simulink model "TEST_IPM_2_0"  (R2019b)
settings: configuration reference "Configuration" (kept outside this file)
PreLoadFcn:
  | RTWConfigurationCB('preloadfcn', bdroot);
values from neighbouring files (symbols this model uses):
  MParamFbase = 200.0    [TEST_IPM_LIB.sldd]
  MParamIbase = 360.0    [TEST_IPM_LIB.sldd]
  MParamLd = 8.0E-5    [TEST_IPM_LIB.sldd]
  MParamLq = 0.00028    [TEST_IPM_LIB.sldd]
  MParamRs = 0.014    [TEST_IPM_LIB.sldd]
  PWM_TPBRD_HALF = 5000.0    [TEST_IPM_LIB.sldd]
  Ts_10kHz = 0.0001    [TEST_IPM_LIB.sldd]
  Ts_1kHz = 0.001    [TEST_IPM_LIB.sldd]
undefined symbols (not defined in the file or in its folder): DiscIntNeverNeededParam, Down, GPTRIP1SEL, GPTRIP2SEL, TZ1, TZ2, Up
libraries: c280xlib x24, c2837xDlib x18, dsparch4 x11, c2802xlib x10, powerlib_meascontrol x9, dspstat3 x2, c2000lib x1, c2806xlib x1, idelinklib_common x1
(part 5 of 6)

== system TEST_IPM_2_0/INT/Motor Control/SVPWM/Inverse Park Transformation ==
  D : Inport
  Q : Inport  Port=2
  theta : Inport  Port=3
  Product{,1..3} (4 alike) : Product  OutDataTypeStr=Inherit: Same as first input
  Sin : Trigonometry  OutputSignalType=real
  Sin1 : Trigonometry  Operator=cos  OutputSignalType=real
  Sum1 : Sum  Inputs=|++  OutDataTypeStr=Inherit: Same as first input
  Sum2 : Sum  Inputs=|+-  OutDataTypeStr=Inherit: Same as first input
  Alpha : Outport
  Beta : Outport  Port=2
  wires:
  Sin1/1 -> Product2/2, Product/2
  Sin/1 -> Product3/2, Product1/2
  Product3/1 -> Sum1/2
  Sum1/1 -> Beta/1
  D/1 -> Product3/1, Product/1
  Product2/1 -> Sum1/1
  Sum2/1 -> Alpha/1
  Product/1 -> Sum2/1
  Product1/1 -> Sum2/2
  Q/1 -> Product2/1, Product1/1
  theta/1 -> Sin/1, Sin1/1

== system TEST_IPM_2_0/INT/Motor Control/SpeedMode/Function-Call Subsystem ==
  function : TriggerPort  TriggerType=function-call  VariantControl=Variant
  Abs : Abs  Commented=on  OutDataTypeStr=single
  Constant : Constant  Value=0  OutDataTypeStr=single  SampleTime=-1
  Constant1 : Constant  Value=0  OutDataTypeStr=single  SampleTime=-1
  Constant2 : Constant  Value=0  OutDataTypeStr=single
  Data Store Read1 : DataStoreRead  DataStoreName=N_FBK
  Data Store Read2 : DataStoreRead  DataStoreName=STOP
  Data Store Read3 : DataStoreRead  DataStoreName=N_REF
  Data Store Write1 : DataStoreWrite  DataStoreName=Iq_REF
  Data Store Write2 : DataStoreWrite  DataStoreName=Id_REF
  Demux : Demux  Outputs=2
  Gain : Gain  Commented=on  Gain=-0.5  OutDataTypeStr=single
  Gain1 : Gain  Commented=on  Gain=0.866  OutDataTypeStr=single
  Mux : Mux  Inputs=2
  Mux1 : Mux  Inputs=2
  "PID_n " : Subsystem
  Switch : Switch  Criteria=u2 ~= 0
  wires:
  Constant/1 -> Mux1/1
  Constant1/1 -> Mux1/2
  Switch/1 -> Demux/1
  Data Store Read1/1 -> Mux/2
  Demux/2 -> "PID_n "/2(Fbk)
  Demux/1 -> "PID_n "/1(Ref)
  Mux1/1 -> Switch/1
  Data Store Read2/1 -> Switch/2
  Data Store Read3/1 -> Mux/1
  Mux/1 -> Switch/3
  "PID_n "/1(Out) -> Data Store Write1/1, Abs/1
  Abs/1 -> Gain/1
  Constant2/1 -> Data Store Write2/1

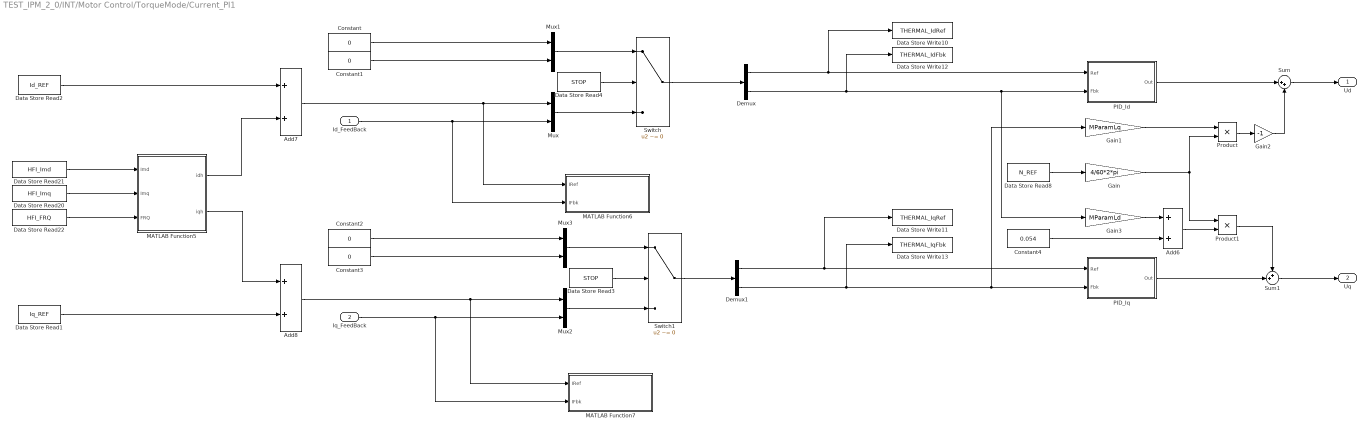
== system TEST_IPM_2_0/INT/Motor Control/TorqueMode/Current_PI1 ==
  Id_FeedBack : Inport
  Iq_FeedBack : Inport  Port=2
  Add6 : Sum
  Add7 : Sum
  Add8 : Sum
  Constant{,1..3} (4 alike) : Constant  Value=0  OutDataTypeStr=single  SampleTime=-1
  Constant4 : Constant  Value=0.054  OutDataTypeStr=single  SampleTime=-1
  Data Store Read1 : DataStoreRead  DataStoreName=Iq_REF
  Data Store Read2 : DataStoreRead  DataStoreName=Id_REF
  Data Store Read20 : DataStoreRead  DataStoreName=HFI_Imq
  Data Store Read21 : DataStoreRead  DataStoreName=HFI_Imd
  Data Store Read22 : DataStoreRead  DataStoreName=HFI_FRQ
  Data Store Read3 : DataStoreRead  DataStoreName=STOP
  Data Store Read4 : DataStoreRead  DataStoreName=STOP
  Data Store Read8 : DataStoreRead  DataStoreName=N_REF
  Data Store Write10 : DataStoreWrite  DataStoreName=THERMAL_IdRef
  Data Store Write11 : DataStoreWrite  DataStoreName=THERMAL_IqRef
  Data Store Write12 : DataStoreWrite  DataStoreName=THERMAL_IdFbk
  Data Store Write13 : DataStoreWrite  DataStoreName=THERMAL_IqFbk
  Demux : Demux  Outputs=2
  Demux1 : Demux  Outputs=2
  Gain : Gain  Gain=4/60*2*pi
  Gain1 : Gain  Gain=MParamLq
  Gain2 : Gain  Gain=-1
  Gain3 : Gain  Gain=MParamLd
  MATLAB Function5 : MATLAB Function  TreatAsAtomicUnit=on
  MATLAB Function6 : MATLAB Function  TreatAsAtomicUnit=on
  MATLAB Function7 : MATLAB Function  TreatAsAtomicUnit=on
  Mux{,1..3} (4 alike) : Mux  Inputs=2
  "PID_Id " : Subsystem  TreatAsAtomicUnit=on
  PID_Iq : Subsystem  TreatAsAtomicUnit=on
  Product : Product
  Product1 : Product
  Sum : Sum  Inputs=|++  AccumDataTypeStr=single
  Sum1 : Sum  Inputs=++|  AccumDataTypeStr=single
  Switch : Switch  Criteria=u2 ~= 0
  Switch1 : Switch  Criteria=u2 ~= 0
  Ud : Outport
  Uq : Outport  Port=2
  wires:
  Demux1/2 -> Data Store Write13/1, Gain1/1, PID_Iq/2(Fbk)
  Demux/1 -> Data Store Write10/1, "PID_Id "/1(Ref)
  Data Store Read1/1 -> Add8/2
  Add8/1 -> MATLAB Function7/1(IRef), Mux2/1
  Constant3/1 -> Mux3/2
  Gain2/1 -> Sum/2
  "PID_Id "/1(Out) -> Sum/1
  Gain/1 -> Product1/1, Product/2
  Switch/1 -> Demux/1
  Data Store Read21/1 -> MATLAB Function5/1(Imd)
  Mux3/1 -> Switch1/1
  Switch1/1 -> Demux1/1
  Gain3/1 -> Add6/1
  Mux/1 -> Switch/3
  Data Store Read3/1 -> Switch1/2
  Iq_FeedBack/1 -> MATLAB Function7/2(IFbk), Mux2/2
  Add6/1 -> Product1/2
  Gain1/1 -> Product/1
  Mux2/1 -> Switch1/3
  Data Store Read8/1 -> Gain/1
  Constant2/1 -> Mux3/1
  MATLAB Function5/1(idh) -> Add7/2
  MATLAB Function5/2(iqh) -> Add8/1
  Data Store Read20/1 -> MATLAB Function5/2(Imq)
  Constant1/1 -> Mux1/2
  Product1/1 -> Sum1/1
  Mux1/1 -> Switch/1
  Data Store Read4/1 -> Switch/2
  Constant4/1 -> Add6/2
  Add7/1 -> MATLAB Function6/1(IRef), Mux/1
  Data Store Read2/1 -> Add7/1
  PID_Iq/1(Out) -> Sum1/2
  Data Store Read22/1 -> MATLAB Function5/3(FRQ)
  Constant/1 -> Mux1/1
  Id_FeedBack/1 -> MATLAB Function6/2(IFbk), Mux/2
  Demux/2 -> Data Store Write12/1, Gain3/1, "PID_Id "/2(Fbk)
  Demux1/1 -> Data Store Write11/1, PID_Iq/1(Ref)
  Product/1 -> Gain2/1
  Sum/1 -> Ud/1
  Sum1/1 -> Uq/1

== system TEST_IPM_2_0/INT/Motor Control/TorqueMode/Function-Call Subsystem ==
  function : TriggerPort  TriggerType=function-call  VariantControl=Variant
  Constant : Constant  Value=0  OutDataTypeStr=single  SampleTime=-1
  Constant1 : Constant  Value=0  OutDataTypeStr=single  SampleTime=-1
  Constant2 : Constant  Value=0  OutDataTypeStr=single  SampleTime=-1
  Constant3 : Constant  OutDataTypeStr=uint16  SampleTime=-1
  Data Store Write : DataStoreWrite  DataStoreName=N_Integral
  Data Store Write1 : DataStoreWrite  DataStoreName=Iq_Integral
  Data Store Write2 : DataStoreWrite  DataStoreName=Id_Integral
  Data Store Write3 : DataStoreWrite  DataStoreName=REVERSE_FLAG
  wires:
  Constant1/1 -> Data Store Write2/1
  Constant2/1 -> Data Store Write1/1
  Constant/1 -> Data Store Write/1
  Constant3/1 -> Data Store Write3/1

== system TEST_IPM_2_0/INT/Motor Control/TorqueMode/PID_n  ==
  Ref : Inport
  Fbk : Inport  Port=2
  Constant : Constant  Value=40*1.2  OutDataTypeStr=single  SampleTime=-1
  Data Store Read : DataStoreRead  DataStoreName=Udc_Integral
  Data Store Read2 : DataStoreRead  DataStoreName=Udc_Kp
  Data Store Write1 : DataStoreWrite  DataStoreName=Udc_Integral
  MATLAB Function : MATLAB Function  TreatAsAtomicUnit=on
  Product : Product  OutDataTypeStr=Inherit: Same as first input
  Subsystem : Subsystem
  Sum1 : Sum  OutDataTypeStr=single
  Sum2 : Sum  Inputs=+-  OutDataTypeStr=Inherit: Inherit via back propagation
  Out : Outport
  wires:
  Data Store Read/1 -> Subsystem/1(OLD_UI_REG3)
  Fbk/1 -> Sum2/2
  Ref/1 -> Sum2/1
  Product/1 -> Sum1/1
  Data Store Read2/1 -> Product/2
  Subsystem/1(UI_REG1) -> Data Store Write1/1, Sum1/2
  Sum2/1 -> Subsystem/2(up_reg3), Product/1
  MATLAB Function/1(Output) -> Out/1
  Sum1/1 -> MATLAB Function/2(Input)
  Constant/1 -> MATLAB Function/1(Limit)

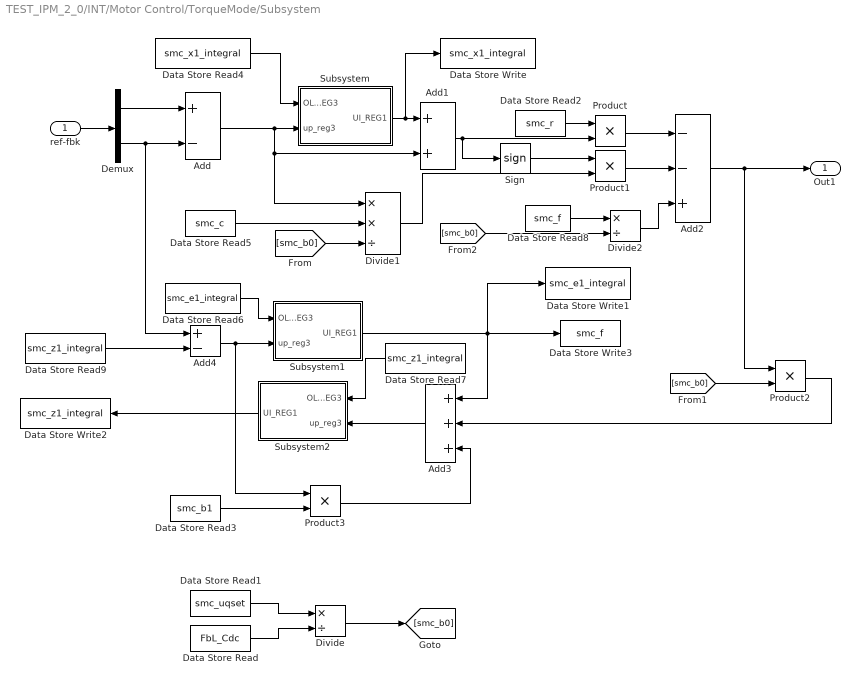
== system TEST_IPM_2_0/INT/Motor Control/TorqueMode/Subsystem ==
  ref-fbk : Inport
  Add : Sum  Inputs=+-
  Add1 : Sum
  Add2 : Sum  Inputs=--+
  Add3 : Sum  Inputs=+++
  Add4 : Sum  Inputs=+-
  Data Store Read : DataStoreRead  DataStoreName=FbL_Cdc
  Data Store Read1 : DataStoreRead  DataStoreName=smc_uqset
  Data Store Read2 : DataStoreRead  DataStoreName=smc_r
  Data Store Read3 : DataStoreRead  DataStoreName=smc_b1
  Data Store Read4 : DataStoreRead  DataStoreName=smc_x1_integral
  Data Store Read5 : DataStoreRead  DataStoreName=smc_c
  Data Store Read6 : DataStoreRead  DataStoreName=smc_e1_integral
  Data Store Read7 : DataStoreRead  DataStoreName=smc_z1_integral
  Data Store Read8 : DataStoreRead  DataStoreName=smc_f
  Data Store Read9 : DataStoreRead  DataStoreName=smc_z1_integral
  Data Store Write : DataStoreWrite  DataStoreName=smc_x1_integral
  Data Store Write1 : DataStoreWrite  DataStoreName=smc_e1_integral
  Data Store Write2 : DataStoreWrite  DataStoreName=smc_z1_integral
  Data Store Write3 : DataStoreWrite  DataStoreName=smc_f
  Demux : Demux  Outputs=2
  Divide : Product  Inputs=*/
  Divide1 : Product  Inputs=**/
  Divide2 : Product  Inputs=*/
  Product{,1..3} (4 alike) : Product
  Sign : Signum
  Subsystem : Subsystem
  Subsystem1 : Subsystem
  Subsystem2 : Subsystem
  Out1 : Outport
  wires:
  ref-fbk/1 -> Demux/1
  Demux/1 -> Add/1
  Demux/2 -> Add4/1, Add/2
  Add/1 -> Divide1/1, Add1/2, Subsystem/2(up_reg3)
  Subsystem/1(UI_REG1) -> Data Store Write/1, Add1/1
  Add1/1 -> Product/2, Sign/1
  Data Store Read2/1 -> Product/1
  Product/1 -> Add2/1
  Product1/1 -> Add2/2
  Sign/1 -> Product1/1
  Data Store Read1/1 -> Divide/1
  Data Store Read/1 -> Divide/2
  Divide/1 -> [smc_b0]
  Data Store Read5/1 -> Divide1/2
  [smc_b0] -> Divide1/3
  Divide1/1 -> Product1/2
  Add2/1 -> Out1/1, Product2/1
  [smc_b0] -> Product2/2
  [smc_b0] -> Divide2/2
  Divide2/1 -> Add2/3
  Add4/1 -> Subsystem1/2(up_reg3), Product3/1
  Subsystem1/1(UI_REG1) -> Data Store Write1/1, Data Store Write3/1, Add3/1
  Product2/1 -> Add3/2
  Add3/1 -> Subsystem2/2(up_reg3)
  Subsystem2/1(UI_REG1) -> Data Store Write2/1
  Data Store Read3/1 -> Product3/2
  Product3/1 -> Add3/3
  Data Store Read4/1 -> Subsystem/1(OLD_UI_REG3)
  Data Store Read6/1 -> Subsystem1/1(OLD_UI_REG3)
  Data Store Read7/1 -> Subsystem2/1(OLD_UI_REG3)
  Data Store Read8/1 -> Divide2/1
  Data Store Read9/1 -> Add4/2

== system TEST_IPM_2_0/INT/Motor Control/VF/Subsystem1 ==
  TargetValue : Inport
  Step : Inport  Port=2
  MATLAB Function : MATLAB Function  TreatAsAtomicUnit=on
  Unit Delay : UnitDelay  SampleTime=-1  HasFrameUpgradeWarning=on
  RampOutput : Outport
  wires:
  TargetValue/1 -> MATLAB Function/1(Target)
  MATLAB Function/1(Output) -> RampOutput/1, Unit Delay/1
  Step/1 -> MATLAB Function/2(Step)
  Unit Delay/1 -> MATLAB Function/3(LastOutput)

== system TEST_IPM_2_0/INT/Motor Control/VF/Subsystem2 ==
  FRQ : Inport
  MATLAB Function : MATLAB Function  TreatAsAtomicUnit=on
  Unit Delay : UnitDelay  SampleTime=-1  HasFrameUpgradeWarning=on
  Ang : Outport
  wires:
  MATLAB Function/1(Ang) -> Ang/1, Unit Delay/1
  Unit Delay/1 -> MATLAB Function/2(LastAng)
  FRQ/1 -> MATLAB Function/1(FRQ)

== system TEST_IPM_2_0/INT/Read Rotor Position/SpeedCal/First Order Filter  ==
  input : Inport
  Add : Sum  Inputs=+-
  Add3 : Sum  AccumDataTypeStr=single
  Constant : Constant  OutDataTypeStr=single  SampleTime=-1
  Data Store Read1 : DataStoreRead  DataStoreName=N_Filter
  Data Store Read2 : DataStoreRead  DataStoreName=N_Filter
  Gain : Gain  Gain=2*pi*Ts_1kHz
  Gain1 : Gain  Gain=2*pi*Ts_1kHz
  Product : Product
  Product1 : Product
  Unit Delay3 : UnitDelay  SampleTime=-1  HasFrameUpgradeWarning=on
  "output " : Outport
  wires:
  input/1 -> Product/1
  Product/1 -> Add3/1
  Product1/1 -> Unit Delay3/1
  Add3/1 -> Product1/1, "output "/1
  Unit Delay3/1 -> Add3/2
  Data Store Read2/1 -> Gain/1
  Gain/1 -> Product/2
  Data Store Read1/1 -> Gain1/1
  Add/1 -> Product1/2
  Gain1/1 -> Add/2
  Constant/1 -> Add/1

== system TEST_IPM_2_0/INT/Motor Control/Current_PI/DEKF_Filter/Subsystem ==
  "InputSignal " : Inport
  "Frq " : Inport  Port=2
  K : Inport  Port=3
  Add : Sum  Inputs=-+
  Add1 : Sum  Inputs=+-
  Add2 : Sum  Inputs=+-
  Discrete-Time Integrator : DiscreteIntegrator  SampleTime=-1  ICPrevOutput=DiscIntNeverNeededParam  ICPrevScaledInput=DiscIntNeverNeededParam
  Discrete-Time Integrator1 : DiscreteIntegrator  SampleTime=-1  ICPrevOutput=DiscIntNeverNeededParam  ICPrevScaledInput=DiscIntNeverNeededParam
  Gain1 : Gain  Gain=2*pi
  Product : Product
  Product1 : Product
  Product2 : Product
  OutputSignal : Outport
  OutputSignal90Deg : Outport  Port=2
  BandStopSignal : Outport  Port=3
  wires:
  Product2/1 -> Add1/1
  "InputSignal "/1 -> Add2/2, Add/2
  Discrete-Time Integrator/1 -> Add2/1, Product1/2, Add/1, OutputSignal/1
  "Frq "/1 -> Gain1/1
  Product1/1 -> Discrete-Time Integrator1/1
  Discrete-Time Integrator1/1 -> OutputSignal90Deg/1, Add1/2
  Product/1 -> Discrete-Time Integrator/1
  Add1/1 -> Product/1
  Add/1 -> Product2/2
  Gain1/1 -> Product/2, Product1/1
  K/1 -> Product2/1
  Add2/1 -> BandStopSignal/1

== system TEST_IPM_2_0/INT/Motor Control/Current_PI/DEKF_Filter/Subsystem1 ==
  "InputSignal " : Inport
  "Frq " : Inport  Port=2
  K : Inport  Port=3
  Add : Sum  Inputs=-+
  Add1 : Sum  Inputs=+-
  Add2 : Sum  Inputs=+-
  Discrete-Time Integrator : DiscreteIntegrator  SampleTime=-1  ICPrevOutput=DiscIntNeverNeededParam  ICPrevScaledInput=DiscIntNeverNeededParam
  Discrete-Time Integrator1 : DiscreteIntegrator  SampleTime=-1  ICPrevOutput=DiscIntNeverNeededParam  ICPrevScaledInput=DiscIntNeverNeededParam
  Gain1 : Gain  Gain=2*pi
  Product : Product
  Product1 : Product
  Product2 : Product
  OutputSignal : Outport
  OutputSignal90Deg : Outport  Port=2
  BandStopSignal : Outport  Port=3
  wires:
  Add2/1 -> BandStopSignal/1
  K/1 -> Product2/1
  Gain1/1 -> Product1/1, Product/2
  Add/1 -> Product2/2
  Add1/1 -> Product/1
  Product/1 -> Discrete-Time Integrator/1
  Discrete-Time Integrator1/1 -> Add1/2, OutputSignal90Deg/1
  Product1/1 -> Discrete-Time Integrator1/1
  "Frq "/1 -> Gain1/1
  Discrete-Time Integrator/1 -> OutputSignal/1, Add/1, Product1/2, Add2/1
  "InputSignal "/1 -> Add/2, Add2/2
  Product2/1 -> Add1/1

== system TEST_IPM_2_0/INT/Motor Control/Current_PI/DEKF_Filter/Subsystem2 ==
  "InputSignal " : Inport
  "Frq " : Inport  Port=2
  K : Inport  Port=3
  Add : Sum  Inputs=-+
  Add1 : Sum  Inputs=+-
  Add2 : Sum  Inputs=+-
  Discrete-Time Integrator : DiscreteIntegrator  SampleTime=-1  ICPrevOutput=DiscIntNeverNeededParam  ICPrevScaledInput=DiscIntNeverNeededParam
  Discrete-Time Integrator1 : DiscreteIntegrator  SampleTime=-1  ICPrevOutput=DiscIntNeverNeededParam  ICPrevScaledInput=DiscIntNeverNeededParam
  Gain1 : Gain  Gain=2*pi
  Product : Product
  Product1 : Product
  Product2 : Product
  OutputSignal : Outport
  OutputSignal90Deg : Outport  Port=2
  BandStopSignal : Outport  Port=3
  wires:
  Add2/1 -> BandStopSignal/1
  K/1 -> Product2/1
  Gain1/1 -> Product1/1, Product/2
  Add/1 -> Product2/2
  Add1/1 -> Product/1
  Product/1 -> Discrete-Time Integrator/1
  Discrete-Time Integrator1/1 -> Add1/2, OutputSignal90Deg/1
  Product1/1 -> Discrete-Time Integrator1/1
  "Frq "/1 -> Gain1/1
  Discrete-Time Integrator/1 -> OutputSignal/1, Add/1, Product1/2, Add2/1
  "InputSignal "/1 -> Add/2, Add2/2
  Product2/1 -> Add1/1

== system TEST_IPM_2_0/INT/Motor Control/Current_PI/DEKF_Filter/Subsystem3 ==
  "InputSignal " : Inport
  "Frq " : Inport  Port=2
  K : Inport  Port=3
  Add : Sum  Inputs=-+
  Add1 : Sum  Inputs=+-
  Add2 : Sum  Inputs=+-
  Discrete-Time Integrator : DiscreteIntegrator  SampleTime=-1  ICPrevOutput=DiscIntNeverNeededParam  ICPrevScaledInput=DiscIntNeverNeededParam
  Discrete-Time Integrator1 : DiscreteIntegrator  SampleTime=-1  ICPrevOutput=DiscIntNeverNeededParam  ICPrevScaledInput=DiscIntNeverNeededParam
  Gain1 : Gain  Gain=2*pi
  Product : Product
  Product1 : Product
  Product2 : Product
  OutputSignal : Outport
  OutputSignal90Deg : Outport  Port=2
  BandStopSignal : Outport  Port=3
  wires:
  Product2/1 -> Add1/1
  "InputSignal "/1 -> Add2/2, Add/2
  Discrete-Time Integrator/1 -> Add2/1, Product1/2, Add/1, OutputSignal/1
  "Frq "/1 -> Gain1/1
  Product1/1 -> Discrete-Time Integrator1/1
  Discrete-Time Integrator1/1 -> OutputSignal90Deg/1, Add1/2
  Product/1 -> Discrete-Time Integrator/1
  Add1/1 -> Product/1
  Add/1 -> Product2/2
  Gain1/1 -> Product/2, Product1/1
  K/1 -> Product2/1
  Add2/1 -> BandStopSignal/1

== system TEST_IPM_2_0/INT/Motor Control/Current_PI/RealVoltageCompesation /Clark Transformation ==
  U : Inport
  V : Inport  Port=2
  W : Inport  Port=3
  Add : Sum  Inputs=+--
  Add1 : Sum  Inputs=+-
  Gain : Gain  Gain=0.5
  Gain1 : Gain  Gain=0.5
  Gain2 : Gain  Gain=2/3
  Gain3 : Gain  Gain=2/3*0.86602540
  Alpha : Outport
  Beta : Outport  Port=2
  wires:
  V/1 -> Add1/1, Gain/1
  Gain/1 -> Add/2
  W/1 -> Add1/2, Gain1/1
  Gain1/1 -> Add/3
  U/1 -> Add/1
  Add/1 -> Gain2/1
  Gain2/1 -> Alpha/1
  Add1/1 -> Gain3/1
  Gain3/1 -> Beta/1

== system TEST_IPM_2_0/INT/Motor Control/Current_PI/RealVoltageCompesation /Park Transformation ==
  Alpha : Inport
  Beta : Inport  Port=2
  theta : Inport  Port=3
  Add : Sum
  Add1 : Sum  Inputs=+-
  Product{,1..3} (4 alike) : Product
  Sin : Trigonometry  OutputSignalType=real
  Sin1 : Trigonometry  Operator=cos  OutputSignalType=real
  D : Outport
  Q : Outport  Port=2
  wires:
  Product/1 -> Add/1
  Sin/1 -> Product3/2, Product1/2
  Product1/1 -> Add/2
  Add1/1 -> Q/1
  Sin1/1 -> Product2/2, Product/2
  Product2/1 -> Add1/1
  Alpha/1 -> Product3/1, Product/1
  Beta/1 -> Product2/1, Product1/1
  Product3/1 -> Add1/2
  Add/1 -> D/1
  theta/1 -> Sin/1, Sin1/1

== system TEST_IPM_2_0/INT/Motor Control/Current_PI/RealVoltageCompesation /Park Transformation1 ==
  Alpha : Inport
  Beta : Inport  Port=2
  theta : Inport  Port=3
  Add : Sum
  Add1 : Sum  Inputs=+-
  Product{,1..3} (4 alike) : Product
  Sin : Trigonometry  OutputSignalType=real
  Sin1 : Trigonometry  Operator=cos  OutputSignalType=real
  D : Outport
  Q : Outport  Port=2
  wires:
  theta/1 -> Sin1/1, Sin/1
  Add/1 -> D/1
  Product3/1 -> Add1/2
  Beta/1 -> Product1/1, Product2/1
  Alpha/1 -> Product/1, Product3/1
  Product2/1 -> Add1/1
  Sin1/1 -> Product/2, Product2/2
  Add1/1 -> Q/1
  Product1/1 -> Add/2
  Sin/1 -> Product1/2, Product3/2
  Product/1 -> Add/1

== system TEST_IPM_2_0/INT/Motor Control/Current_PI/deadzone compesation/Clark Transformation ==
  U : Inport
  V : Inport  Port=2
  W : Inport  Port=3
  Add : Sum  Inputs=+--
  Add1 : Sum  Inputs=+-
  Gain : Gain  Gain=0.5
  Gain1 : Gain  Gain=0.5
  Gain2 : Gain  Gain=2/3
  Gain3 : Gain  Gain=2/3*0.86602540
  Alpha : Outport
  Beta : Outport  Port=2
  wires:
  V/1 -> Add1/1, Gain/1
  Gain/1 -> Add/2
  W/1 -> Add1/2, Gain1/1
  Gain1/1 -> Add/3
  U/1 -> Add/1
  Add/1 -> Gain2/1
  Gain2/1 -> Alpha/1
  Add1/1 -> Gain3/1
  Gain3/1 -> Beta/1

== system TEST_IPM_2_0/INT/Motor Control/Current_PI/deadzone compesation/Park Transformation ==
  Alpha : Inport
  Beta : Inport  Port=2
  theta : Inport  Port=3
  Add : Sum
  Add1 : Sum  Inputs=+-
  Product{,1..3} (4 alike) : Product
  Sin : Trigonometry  OutputSignalType=real
  Sin1 : Trigonometry  Operator=cos  OutputSignalType=real
  D : Outport
  Q : Outport  Port=2
  wires:
  Product/1 -> Add/1
  Sin/1 -> Product3/2, Product1/2
  Product1/1 -> Add/2
  Add1/1 -> Q/1
  Sin1/1 -> Product2/2, Product/2
  Product2/1 -> Add1/1
  Alpha/1 -> Product3/1, Product/1
  Beta/1 -> Product2/1, Product1/1
  Product3/1 -> Add1/2
  Add/1 -> D/1
  theta/1 -> Sin/1, Sin1/1

== system TEST_IPM_2_0/INT/Motor Control/FbLMode/Subsystem/PID_z1  ==
  Ref : Inport
  Fbk : Inport  Port=2
  Data Store Read : DataStoreRead  DataStoreName=FbL_z1_Integral
  Data Store Read4 : DataStoreRead  DataStoreName=FbL_k1
  Data Store Write : DataStoreWrite  DataStoreName=FbL_z1_Integral
  Gain : Gain  Gain=-1e-4  OutDataTypeStr=single
  Product : Product  OutDataTypeStr=Inherit: Same as first input
  Subsystem : Subsystem
  Sum1 : Sum  OutDataTypeStr=single
  Sum2 : Sum  Inputs=-+  OutDataTypeStr=Inherit: Inherit via back propagation
  Out : Outport
  wires:
  Subsystem/1(UI_REG1) -> Data Store Write/1, Sum1/2
  Fbk/1 -> Sum2/2
  Ref/1 -> Sum2/1
  Product/1 -> Sum1/1
  Data Store Read4/1 -> Gain/1
  Sum2/1 -> Subsystem/2(up_reg3), Product/1
  Sum1/1 -> Out/1
  Gain/1 -> Product/2
  Data Store Read/1 -> Subsystem/1(OLD_UI_REG3)

== system TEST_IPM_2_0/INT/Motor Control/FbLMode/Subsystem/PID_z3 ==
  Ref : Inport
  Fbk : Inport  Port=2
  Data Store Read : DataStoreRead  DataStoreName=FbL_z3_Integral
  Data Store Read1 : DataStoreRead  DataStoreName=FbL_k5
  Data Store Write1 : DataStoreWrite  DataStoreName=FbL_z3_Integral
  Gain : Gain  Gain=-1e-4  OutDataTypeStr=single
  Product : Product  OutDataTypeStr=Inherit: Same as first input
  Subsystem : Subsystem
  Sum1 : Sum  OutDataTypeStr=single
  Sum2 : Sum  Inputs=-+  OutDataTypeStr=Inherit: Inherit via back propagation
  Out : Outport
  wires:
  Gain/1 -> Product/2
  Sum1/1 -> Out/1
  Sum2/1 -> Product/1, Subsystem/2(up_reg3)
  Product/1 -> Sum1/1
  Ref/1 -> Sum2/1
  Fbk/1 -> Sum2/2
  Subsystem/1(UI_REG1) -> Data Store Write1/1, Sum1/2
  Data Store Read1/1 -> Gain/1
  Data Store Read/1 -> Subsystem/1(OLD_UI_REG3)

== system TEST_IPM_2_0/INT/Motor Control/FbLMode/Subsystem/Subsystem ==
  z2 : Inport
  z1ref : Inport  Port=2
  z1 : Inport  Port=3
  Add : Sum  Inputs=+-
  Add1 : Sum  Inputs=+++
  Add2 : Sum
  Data Store Read : DataStoreRead  DataStoreName=FbL_smc_integral
  Data Store Read1 : DataStoreRead  DataStoreName=FbL_smc_r1
  Data Store Read2 : DataStoreRead  DataStoreName=FbL_smc_r2
  Data Store Write : DataStoreWrite  DataStoreName=FbL_smc_integral
  Gain : Gain  Gain=600
  Product : Product
  Product1 : Product
  Sign : Signum
  Subsystem : Subsystem
  Out1 : Outport
  wires:
  z1/1 -> Add/1
  z1ref/1 -> Add/2
  Add/1 -> Subsystem/2(up_reg3), Gain/1
  Data Store Read/1 -> Subsystem/1(OLD_UI_REG3)
  Subsystem/1(UI_REG1) -> Add1/1, Data Store Write/1
  Gain/1 -> Add1/2
  z2/1 -> Add1/3
  Add1/1 -> Sign/1, Product/1
  Data Store Read1/1 -> Product/2
  Sign/1 -> Product1/1
  Data Store Read2/1 -> Product1/2
  Product/1 -> Add2/1
  Product1/1 -> Add2/2
  Add2/1 -> Out1/1

== system TEST_IPM_2_0/INT/Motor Control/SpeedMode/Function-Call Subsystem/PID_n  ==
  Ref : Inport
  Fbk : Inport  Port=2
  Constant : Constant  Value=MParamIbase*1.2  OutDataTypeStr=single  SampleTime=-1
  Data Store Read : DataStoreRead  DataStoreName=N_Kp
  Data Store Read1 : DataStoreRead  DataStoreName=N_Integral
  Data Store Write : DataStoreWrite  DataStoreName=N_Integral
  MATLAB Function : MATLAB Function  TreatAsAtomicUnit=on
  Product : Product  OutDataTypeStr=Inherit: Same as first input
  Subsystem : Subsystem
  Sum1 : Sum  OutDataTypeStr=single
  Sum2 : Sum  Inputs=+-  OutDataTypeStr=Inherit: Inherit via back propagation
  Out : Outport
  wires:
  Data Store Read1/1 -> Subsystem/1(OLD_UI_REG3)
  Fbk/1 -> Sum2/2
  Ref/1 -> Sum2/1
  Product/1 -> Sum1/1
  Data Store Read/1 -> Product/2
  Subsystem/1(UI_REG1) -> Data Store Write/1, Sum1/2
  Sum2/1 -> Subsystem/2(up_reg3), Product/1
  MATLAB Function/1(Output) -> Out/1
  Sum1/1 -> MATLAB Function/2(Input)
  Constant/1 -> MATLAB Function/1(Limit)

== system TEST_IPM_2_0/INT/Motor Control/TorqueMode/Current_PI1/PID_Id  ==
  Ref : Inport
  Fbk : Inport  Port=2
  Data Store Read : DataStoreRead  DataStoreName=Id_Kp
  Data Store Read1 : DataStoreRead  DataStoreName=Id_Integral
  Data Store Read3 : DataStoreRead  DataStoreName=UDCPROTECT
  Data Store Write : DataStoreWrite  DataStoreName=Id_Integral
  MATLAB Function1 : MATLAB Function  TreatAsAtomicUnit=on
  Product : Product  OutDataTypeStr=Inherit: Same as first input
  Subsystem : Subsystem
  Sum1 : Sum  OutDataTypeStr=single
  Sum2 : Sum  Inputs=+-  OutDataTypeStr=Inherit: Inherit via back propagation
  Out : Outport
  wires:
  Data Store Read1/1 -> Subsystem/1(OLD_UI_REG3)
  Fbk/1 -> Sum2/2
  Ref/1 -> Sum2/1
  Product/1 -> Sum1/1
  Data Store Read/1 -> Product/2
  Sum2/1 -> Subsystem/2(up_reg3), Product/1
  Sum1/1 -> Out/1
  Data Store Read3/1 -> MATLAB Function1/1(Udc)
  Subsystem/1(UI_REG1) -> MATLAB Function1/2(Input), Sum1/2
  MATLAB Function1/1(Output) -> Data Store Write/1

== system TEST_IPM_2_0/INT/Motor Control/TorqueMode/Current_PI1/PID_Iq ==
  Ref : Inport
  Fbk : Inport  Port=2
  Data Store Read : DataStoreRead  DataStoreName=Iq_Kp
  Data Store Read1 : DataStoreRead  DataStoreName=Iq_Integral
  Data Store Read2 : DataStoreRead  DataStoreName=UDCPROTECT
  Data Store Read3 : DataStoreRead  DataStoreName=UDCPROTECT
  Data Store Write : DataStoreWrite  DataStoreName=Iq_Integral
  MATLAB Function : MATLAB Function  TreatAsAtomicUnit=on
  MATLAB Function1 : MATLAB Function  TreatAsAtomicUnit=on
  Product : Product  OutDataTypeStr=Inherit: Same as first input
  Subsystem : Subsystem
  Sum1 : Sum  OutDataTypeStr=single
  Sum2 : Sum  Inputs=+-  OutDataTypeStr=Inherit: Inherit via back propagation
  Out : Outport
  wires:
  MATLAB Function1/1(Output) -> Data Store Write/1
  Subsystem/1(UI_REG1) -> Sum1/2, MATLAB Function1/2(Input)
  Data Store Read3/1 -> MATLAB Function1/1(Udc)
  MATLAB Function/1(Output) -> Out/1
  Data Store Read2/1 -> MATLAB Function/1(Udc)
  Sum1/1 -> MATLAB Function/2(Input)
  Sum2/1 -> Product/1, Subsystem/2(up_reg3)
  Data Store Read/1 -> Product/2
  Product/1 -> Sum1/1
  Ref/1 -> Sum2/1
  Fbk/1 -> Sum2/2
  Data Store Read1/1 -> Subsystem/1(OLD_UI_REG3)

== system TEST_IPM_2_0/INT/Motor Control/TorqueMode/PID_n /Subsystem ==
  OLD_UI_REG3 : Inport
  up_reg3 : Inport  Port=2
  Data Store Read3 : DataStoreRead  DataStoreName=Udc_Ki
  Gain : Gain  Gain=Ts_10kHz
  Product1 : Product  OutDataTypeStr=Inherit: Same as first input
  Sum3 : Sum  OutDataTypeStr=single
  UI_REG1 : Outport
  wires:
  Sum3/1 -> UI_REG1/1
  up_reg3/1 -> Product1/2
  Product1/1 -> Sum3/2
  OLD_UI_REG3/1 -> Sum3/1
  Gain/1 -> Product1/1
  Data Store Read3/1 -> Gain/1

== system TEST_IPM_2_0/INT/Motor Control/TorqueMode/Subsystem/Subsystem ==
  OLD_UI_REG3 : Inport
  up_reg3 : Inport  Port=2
  Data Store Read1 : DataStoreRead  DataStoreName=smc_c
  Gain : Gain  Gain=Ts_10kHz
  Product1 : Product  OutDataTypeStr=Inherit: Same as first input
  Sum3 : Sum
  UI_REG1 : Outport
  wires:
  Sum3/1 -> UI_REG1/1
  up_reg3/1 -> Product1/2
  Product1/1 -> Sum3/2
  OLD_UI_REG3/1 -> Sum3/1
  Gain/1 -> Product1/1
  Data Store Read1/1 -> Gain/1

== system TEST_IPM_2_0/INT/Motor Control/TorqueMode/Subsystem/Subsystem1 ==
  OLD_UI_REG3 : Inport
  up_reg3 : Inport  Port=2
  Data Store Read : DataStoreRead  DataStoreName=smc_b2
  Gain : Gain  Gain=Ts_10kHz
  Product1 : Product  OutDataTypeStr=Inherit: Same as first input
  Sum3 : Sum
  UI_REG1 : Outport
  wires:
  Data Store Read/1 -> Gain/1
  Gain/1 -> Product1/1
  OLD_UI_REG3/1 -> Sum3/1
  Product1/1 -> Sum3/2
  up_reg3/1 -> Product1/2
  Sum3/1 -> UI_REG1/1

== system TEST_IPM_2_0/INT/Motor Control/TorqueMode/Subsystem/Subsystem2 ==
  OLD_UI_REG3 : Inport
  up_reg3 : Inport  Port=2
  Constant : Constant  OutDataTypeStr=single
  Gain : Gain  Gain=Ts_10kHz
  Product1 : Product  OutDataTypeStr=Inherit: Same as first input
  Sum3 : Sum
  UI_REG1 : Outport
  wires:
  Sum3/1 -> UI_REG1/1
  up_reg3/1 -> Product1/2
  Product1/1 -> Sum3/2
  OLD_UI_REG3/1 -> Sum3/1
  Gain/1 -> Product1/1
  Constant/1 -> Gain/1

== system TEST_IPM_2_0/INT/Motor Control/FbLMode/Subsystem/PID_z1 /Subsystem ==
  OLD_UI_REG3 : Inport
  up_reg3 : Inport  Port=2
  Data Store Read2 : DataStoreRead  DataStoreName=FbL_k0
  Gain : Gain  Gain=Ts_10kHz
  Gain1 : Gain  Gain=-1e-4  OutDataTypeStr=single
  Product1 : Product  OutDataTypeStr=Inherit: Same as first input
  Sum3 : Sum
  UI_REG1 : Outport
  wires:
  Sum3/1 -> UI_REG1/1
  up_reg3/1 -> Product1/2
  Product1/1 -> Sum3/2
  OLD_UI_REG3/1 -> Sum3/1
  Gain/1 -> Product1/1
  Data Store Read2/1 -> Gain1/1
  Gain1/1 -> Gain/1

== system TEST_IPM_2_0/INT/Motor Control/FbLMode/Subsystem/PID_z3/Subsystem ==
  OLD_UI_REG3 : Inport
  up_reg3 : Inport  Port=2
  Data Store Read : DataStoreRead  DataStoreName=FbL_k4
  Gain : Gain  Gain=Ts_10kHz
  Gain1 : Gain  Gain=-1e-4  OutDataTypeStr=single
  Product1 : Product  OutDataTypeStr=Inherit: Same as first input
  Sum3 : Sum
  UI_REG1 : Outport
  wires:
  Gain1/1 -> Gain/1
  Gain/1 -> Product1/1
  OLD_UI_REG3/1 -> Sum3/1
  Product1/1 -> Sum3/2
  up_reg3/1 -> Product1/2
  Sum3/1 -> UI_REG1/1
  Data Store Read/1 -> Gain1/1

== system TEST_IPM_2_0/INT/Motor Control/FbLMode/Subsystem/Subsystem/Subsystem ==
  OLD_UI_REG3 : Inport
  up_reg3 : Inport  Port=2
  Constant : Constant  Value=90000  OutDataTypeStr=single
  Gain : Gain  Gain=Ts_10kHz
  Product1 : Product  OutDataTypeStr=Inherit: Same as first input
  Sum3 : Sum
  UI_REG1 : Outport
  wires:
  Sum3/1 -> UI_REG1/1
  up_reg3/1 -> Product1/2
  Product1/1 -> Sum3/2
  OLD_UI_REG3/1 -> Sum3/1
  Gain/1 -> Product1/1
  Constant/1 -> Gain/1

== system TEST_IPM_2_0/INT/Motor Control/SpeedMode/Function-Call Subsystem/PID_n /Subsystem ==
  OLD_UI_REG3 : Inport
  up_reg3 : Inport  Port=2
  Data Store Read2 : DataStoreRead  DataStoreName=N_Ki
  Gain : Gain  Gain=Ts_1kHz
  Product1 : Product  OutDataTypeStr=Inherit: Same as first input
  Sum3 : Sum  OutDataTypeStr=single
  UI_REG1 : Outport
  wires:
  Sum3/1 -> UI_REG1/1
  up_reg3/1 -> Product1/2
  Product1/1 -> Sum3/2
  OLD_UI_REG3/1 -> Sum3/1
  Gain/1 -> Product1/1
  Data Store Read2/1 -> Gain/1

== system TEST_IPM_2_0/INT/Motor Control/TorqueMode/Current_PI1/PID_Id /Subsystem ==
  OLD_UI_REG3 : Inport
  up_reg3 : Inport  Port=2
  Data Store Read2 : DataStoreRead  DataStoreName=Id_Ki
  Gain : Gain  Gain=Ts_10kHz
  Product1 : Product  OutDataTypeStr=Inherit: Same as first input
  Sum3 : Sum
  UI_REG1 : Outport
  wires:
  Sum3/1 -> UI_REG1/1
  up_reg3/1 -> Product1/2
  Product1/1 -> Sum3/2
  OLD_UI_REG3/1 -> Sum3/1
  Gain/1 -> Product1/1
  Data Store Read2/1 -> Gain/1

== system TEST_IPM_2_0/INT/Motor Control/TorqueMode/Current_PI1/PID_Iq/Subsystem ==
  OLD_UI_REG3 : Inport
  up_reg3 : Inport  Port=2
  Data Store Read2 : DataStoreRead  DataStoreName=Iq_Ki
  Gain : Gain  Gain=Ts_10kHz
  Product1 : Product  OutDataTypeStr=Inherit: Same as first input
  Sum3 : Sum
  UI_REG1 : Outport
  wires:
  Data Store Read2/1 -> Gain/1
  Gain/1 -> Product1/1
  OLD_UI_REG3/1 -> Sum3/1
  Product1/1 -> Sum3/2
  up_reg3/1 -> Product1/2
  Sum3/1 -> UI_REG1/1

== stateflow chart TEST_IPM_2_0/INT/AD2S1210 Init/AD2S1210 ==
  settings: updateMethod=DISCRETE  initializeOutput=1
  state Empty
    entry:
    Wait_Count = 0;
  state RESET_STEP1
    entry:
    Wait_Count  = Wait_Count + 1;
    ResloverRESET = 0;
    EV_RESET();
  state RESET_STEP2
    entry:
    ResloverRESET = 1;
    EV_RESET();
  state INIT_ConfigMode
    entry:
    ResloverA0=1;
    ResloverA1=1;
    ConfigMode();
  state WRITE_FRQ_STEP1
    entry:
    ResloverWR=1;
    WRITE_SPI_STEP1();
  state WRITE_FRQ_STEP4
    entry:
    ResloverWR=1;
    WRITE_SPI_STEP1();
  state READ_FAULT_STEP1
    entry:
    ResloverWR=1;
    WRITE_SPI_STEP1();
  state READ_FAULT_STEP4
    entry:
    ResloverWR=1;
    WRITE_SPI_STEP1();
  state READ_FAULT_STEP5
    entry:
    ResloverWR=1;
    WRITE_SPI_STEP1();
  state WRITE_FRQ_STEP2
    entry:
    ResloverWR=0;
    SPIC_Tx=uint16(hex2dec('9191'));
    WRITE_SPI_STEP2();
  state WRITE_FRQ_STEP5
    entry:
    ResloverWR=0;
    SPIC_Tx=ResloverFRQ*256+ResloverFRQ;
    WRITE_SPI_STEP2();
  state READ_FAULT_STEP2
    entry:
    ResloverWR=0;
    SPIC_Tx=uint16(hex2dec('FFFF'));
    WRITE_SPI_STEP2();
  state READ_FAULT_STEP3
    entry:
    ResloverWR=0;
    SPIC_Tx=uint16(hex2dec('FFFF'));
    WRITE_SPI_STEP2();
  state READ_FAULT_STEP6
    entry:
    ResloverWR=0;
    SPIC_Tx=uint16(hex2dec('FFFF'));
    WRITE_SPI_STEP2();
  state WRITE_RES_STEP1
    entry:
    ResloverWR=1;
    WRITE_SPI_STEP1();
  state WRITE_RES_STEP3
    entry:
    ResloverWR=1;
    WRITE_SPI_STEP1();
  state WRITE_RES_STEP2
    entry:
    ResloverWR=0;
    SPIC_Tx=uint16(hex2dec('9292'));
    WRITE_SPI_STEP2();
  state WRITE_RES_STEP4
    entry:
    ResloverWR=0;
    SPIC_Tx=ResloverRES*256+ResloverRES;
    WRITE_SPI_STEP2();
  state INIT_FINISH
    entry:
    ResloverWR=0;
    ResloverA0=0;
    ResloverA1=0;
    InitMode=2;
    INIT_FINISH();
  (default) -> Empty
  Empty -> RESET_STEP1 : [InitMode==1]
  RESET_STEP1 -> RESET_STEP1 [order 2]
  RESET_STEP1 -> RESET_STEP2 [order 1] : [Wait_Count > 1000]
  INIT_FINISH -> RESET_STEP2
  RESET_STEP2 -> INIT_ConfigMode : [InitMode==1]
  INIT_ConfigMode -> WRITE_FRQ_STEP1
  WRITE_FRQ_STEP2 -> WRITE_FRQ_STEP4
  READ_FAULT_STEP2 -> READ_FAULT_STEP4
  WRITE_RES_STEP4 -> READ_FAULT_STEP1
  READ_FAULT_STEP3 -> READ_FAULT_STEP5
  WRITE_FRQ_STEP1 -> WRITE_FRQ_STEP2
  WRITE_FRQ_STEP4 -> WRITE_FRQ_STEP5
  READ_FAULT_STEP1 -> READ_FAULT_STEP2
  READ_FAULT_STEP4 -> READ_FAULT_STEP3
  READ_FAULT_STEP5 -> READ_FAULT_STEP6
  WRITE_FRQ_STEP5 -> WRITE_RES_STEP1
  READ_FAULT_STEP6 -> INIT_FINISH
  WRITE_RES_STEP2 -> WRITE_RES_STEP3
  WRITE_RES_STEP1 -> WRITE_RES_STEP2
  WRITE_RES_STEP3 -> WRITE_RES_STEP4
  data: ResloverWR data_store_memory; ResloverRESET data_store_memory; SPIC_Tx data_store_memory; ResloverA0 data_store_memory; ResloverA1 data_store_memory; ResloverFRQ data_store_memory; InitMode data_store_memory; ResloverRES data_store_memory; Wait_Count local
  events: EV_RESET output FUNCTION_CALL_EVENT; ConfigMode output FUNCTION_CALL_EVENT; WRITE_SPI_STEP1 output FUNCTION_CALL_EVENT; WRITE_SPI_STEP2 output FUNCTION_CALL_EVENT; INIT_FINISH output FUNCTION_CALL_EVENT

== matlab function TEST_IPM_2_0/INT/Current Bias Init/MATLAB Function ==
  data: InitMode output
function InitMode = TICK_ADD
persistent Tick
if isempty(Tick)
    Tick = uint16(0);
end
Tick = Tick + uint16(1);
if(Tick <= 50000)
    InitMode = uint16(2);
else
    InitMode = uint16(0);
    Tick = uint16(0);
end
end

== stateflow chart TEST_IPM_2_0/INT/Chart ==
  settings: updateMethod=DISCRETE  initializeOutput=1  enableNonTerminalStates=1
  state Empty
  state Init
    entry:
    ADCINT_IN();
  state ADC_Sample
    entry:
    ADCSample();
    ResloverSAMPLE=0;
  state AD2S1210
    entry:
    SPIC_Tx = 0;
    ResloverSAMPLE=1;
    AD2S1210();
  state System_InitADBias
    entry:
    STOP=1;
    INIT_ADBias();
  state System_InitAD2S1210
    entry:
    STOP=1;
    INIT_AD2S1210();
  state MOTORCONTROL
    entry:
    MOTORCONTROL();
  state Extra_Observer
    entry:
    Extra_Observer();
  state ePWM
    entry:
    ePWM();
  state BufferStore
    entry:
    Buffer();
  state DA_5742
    entry:
    DA_5742();
  state end
    entry:
    ADCINT_OUT();
    ChartFlag= 1;
  (default) -> Empty
  end -> Empty
  Empty -> Init : [ChartFlag==0]
  Init -> ADC_Sample
  ADC_Sample -> System_InitAD2S1210 [order 2] : [InitMode==1]
  ADC_Sample -> System_InitADBias [order 3] : [InitMode==2]
  ADC_Sample -> AD2S1210 [order 1] : [InitMode==0]
  AD2S1210 -> MOTORCONTROL
  System_InitAD2S1210 -> ePWM
  System_InitADBias -> ePWM
  MOTORCONTROL -> Extra_Observer [order 2]
  MOTORCONTROL -> ePWM [order 1] : [DEKF_FLAG == 0]
  Extra_Observer -> ePWM
  ePWM -> BufferStore
  BufferStore -> DA_5742
  DA_5742 -> end
  data: InitMode data_store_memory; ChartFlag data_store_memory; ResloverSAMPLE data_store_memory; SPIC_Tx data_store_memory; STOP data_store_memory; DEKF_FLAG data_store_memory
  events: ADCINT_IN output FUNCTION_CALL_EVENT; ADCSample output FUNCTION_CALL_EVENT; INIT_AD2S1210 output FUNCTION_CALL_EVENT; INIT_ADBias output FUNCTION_CALL_EVENT; AD2S1210 output FUNCTION_CALL_EVENT; MOTORCONTROL output FUNCTION_CALL_EVENT; Extra_Observer output FUNCTION_CALL_EVENT; ePWM output FUNCTION_CALL_EVENT; Buffer output FUNCTION_CALL_EVENT; DA_5742 output FUNCTION_CALL_EVENT; ADCINT_OUT output FUNCTION_CALL_EVENT

== matlab function TEST_IPM_2_0/INT/Read Rotor Position/MATLAB Function ==
  events: FunCall output FUNCTION_CALL_EVENT
function SpeedDivder
persistent Tick
if isempty(Tick)
    Tick = uint16(0);
end
Tick = Tick + uint16(1);
if(Tick == 10)
    Tick = uint16(0);
    FunCall;
end

== matlab function TEST_IPM_2_0/INT/Current Sampling/MATLAB Function ==
  data: U input; V input; W input; PROTECT data_store_memory; STOP data_store_memory
function Current_Protect(U,V,W)
global PROTECT STOP
if (U>30||U<-30||V>30||V<-30||W>30||W<-30)
    STOP = uint16(1);
    PROTECT = uint16(bitor(PROTECT,1)); 
end

if(PROTECT ~= uint16(0))
    STOP = uint16(1);
end

== matlab function TEST_IPM_2_0/INT/Motor Control/SpeedMode/MATLAB Function ==
  events: Speed_PI output FUNCTION_CALL_EVENT
function Count()
persistent count; 
if isempty(count)
    count = uint16(0);
end

count = count + uint16(1);
if(count == 10)
    count = uint16(0);
    Speed_PI();
end

end

== matlab function TEST_IPM_2_0/INT/Current Sampling/MATLAB Function1 ==
  data: input input; Output output
function Output = Udc(input)
Output = single((single(input)-single(8))*single(0.147220477)) + single(2.7);
end

== matlab function TEST_IPM_2_0/INT/Read Rotor Position/RAW_DATA2Angle  ==
  data: Raw_Data input; Angle_out output; Mech_Theta_out output; Mid_Position input
function [Angle_out,Mech_Theta_out] = Raw_Data2Angle(Raw_Data,Mid_Position)
    Angle = single(Raw_Data) - single(Mid_Position);
    if(Angle < 0)
        Angle = Angle + single(65535);
    end
    Mech_Theta = single(Angle)*single(1)*(single(1.5259e-5));
    Angle = single(Angle)*single(4)*(single(1.5259e-5));
    Angle = mod(Angle,single(1));
    Mech_Theta = mod(Mech_Theta,single(1));
    Angle_out = Angle;
    Mech_Theta_out = Mech_Theta;
end

== matlab function TEST_IPM_2_0/Temperature&DCBUS/MATLAB Function1 ==
  data: input input; Output output
function Output = Temp(input)
temp_voltage=single(input)*single(0.00073242);
Output = single(126.3) - single(198.8)*temp_voltage + single(133.3)*temp_voltage*temp_voltage-single(33.83)*temp_voltage*temp_voltage*temp_voltage;
end

== matlab function TEST_IPM_2_0/Temperature&DCBUS/MATLAB Function2 ==
  data: input input; Output output
function Output = Temp(input)
temp_voltage=single(input)*single(0.00073242);
Output = single(126.3) - single(198.8)*temp_voltage + single(133.3)*temp_voltage*temp_voltage-single(33.83)*temp_voltage*temp_voltage*temp_voltage;
end

== matlab function TEST_IPM_2_0/Temperature&DCBUS/MATLAB Function3 ==
  data: Temp_Max input; Udc_FBK input; Udc_REF input; N_REF input; N_FBK input; PROTECT data_store_memory; STOP data_store_memory; UDCPROTECT data_store_memory; ControlMode input
function PROTECT(Temp_Max,Udc_FBK,Udc_REF, N_REF,N_FBK,ControlMode)
global PROTECT UDCPROTECT STOP
    if(Temp_Max >= 95)
        PROTECT = uint16(bitor(PROTECT,uint16(4)));
        STOP = uint16(1);
    end
    if(Udc_FBK >= UDCPROTECT + 15 ||Udc_FBK <= UDCPROTECT - 45)
        PROTECT = uint16(bitor(PROTECT,uint16(2)));
        STOP = uint16(1);
    end    

    if((N_FBK >= N_REF + single(300)|| N_FBK<= N_REF - single(300))&&ControlMode==uint16(4))
         PROTECT = uint16(bitor(PROTECT,uint16(8)));
         STOP = uint16(1);
    end
    
    if((Udc_FBK >= Udc_REF + single(15) || Udc_FBK <= Udc_REF - single(15))&&(ControlMode==uint16(3)||ControlMode==uint16(6)))
        PROTECT = uint16(bitor(PROTECT,uint16(4)));
        STOP = uint16(1);
    end
end

== matlab function TEST_IPM_2_0/Temperature&DCBUS/MATLAB Function4 ==
  data: input input; Output output
function Output = Temp(input)
temp_voltage=single(input)*single(0.00073242);
Output = single(126.3) - single(198.8)*temp_voltage + single(133.3)*temp_voltage*temp_voltage-single(33.83)*temp_voltage*temp_voltage*temp_voltage;
end

== matlab function TEST_IPM_2_0/INT/Motor Control/IF/Subsystem1/MATLAB Function ==
  data: Target input single; Output output; Step input single; LastOutput input single
function Output = RAMPCONTROL(Target,Step,LastOutput)
if(LastOutput <= Target)
    Temp = LastOutput + Step;
else
    Temp = LastOutput - Step;
end
if (abs(Temp - Target) <= Step * 2)
    Temp = Target;
end
    Output = Temp;
end

== matlab function TEST_IPM_2_0/INT/Motor Control/SpeedMode/Function-Call Subsystem/PID_n /MATLAB Function ==
  data: Limit input; Input input; Output output
function Output = Saturation(Limit,Input)
if(Input >= Limit)
    Output = Limit;
elseif(Input <= -Limit)
    Output = -Limit;
else
    Output = Input;
end

== matlab function TEST_IPM_2_0/INT/Motor Control/VF/Subsystem1/MATLAB Function ==
  data: Target input single; Output output; Step input single; LastOutput input single
function Output = RAMPCONTROL(Target,Step,LastOutput)
if(LastOutput <= Target)
    Temp = LastOutput + Step;
else
    Temp = LastOutput - Step;
end
if (abs(Temp - Target) <= Step * 2)
    Temp = Target;
end
    Output = Temp;
end

== matlab function TEST_IPM_2_0/INT/Motor Control/SpeedMode/MATLAB Function1 ==
  data: Flag_MTPA input; IqDem input; Id_REF output
function Id_REF = MTPA_Curve(Flag_MTPA,IqDem)
if(Flag_MTPA == uint16(1))
    Id_REF = single(3.8117) -single(0.1816)*IqDem -single(0.0025)*IqDem*IqDem + single(2.3650e-06)*IqDem*IqDem*IqDem;
else
    Id_REF = 0;
end

== matlab function TEST_IPM_2_0/INT/Motor Control/VF/Subsystem2/MATLAB Function ==
  data: FRQ input single; Ang output; LastAng input single
function Ang = AngOutput(FRQ,LastAng)
    Temp = LastAng + FRQ*single(1e-4 * 2* pi);
    if(Temp > single(2*pi))
        Temp = Temp - single(2*pi);
    end
    Ang = Temp;
end

== matlab function TEST_IPM_2_0/INT/Motor Control/IF/Subsystem2/MATLAB Function ==
  data: FRQ input single; Ang output; LastAng input single
function Ang = AngOutput(FRQ,LastAng)
    Temp = LastAng + FRQ*single(1e-4 * 2* pi);
    if(Temp > single(2*pi))
        Temp = Temp - single(2*pi);
    end
    Ang = Temp;
end

== matlab function TEST_IPM_2_0/INT/Motor Control/TorqueMode/Current_PI1/PID_Id /MATLAB Function1 ==
  data: Udc input; Output output; Input input
function Output = Saturation(Udc,Input)
if(Input >= Udc/sqrt(3))
    Output = Udc/sqrt(3);
elseif(Input <= -Udc/sqrt(3))
    Output = -Udc/sqrt(3);
else
    Output = Input;
end

== matlab function TEST_IPM_2_0/INT/Motor Control/Current_PI/MATLAB Function1 ==
  data: Ud input; Uq input; Ud_out output; Us_out output; Uq_out output; ControlMode data_store_memory; VF_Ud data_store_memory; VF_Uq data_store_memory; UDCPROTECT input; STOP data_store_memory
function [Ud_out,Us_out,Uq_out] = Over_Modulation(Ud,Uq,UDCPROTECT)
global ControlMode VF_Ud VF_Uq;
global STOP;
Us = sqrt(Ud*Ud+Uq*Uq);
Us_out = Us;
if(Us>UDCPROTECT/sqrt(3))
    Ud_out_temp = Ud/Us*Ud;
    Uq_out_temp = Uq/Us*Uq;
else
    Ud_out_temp = Ud;
    Uq_out_temp = Uq;
end
    
if(ControlMode == 1)
    Ud_out = VF_Ud;
    Uq_out = VF_Uq;
else
    Ud_out = Ud_out_temp;
    Uq_out = Uq_out_temp;
end

if(STOP ~= 0)
    Ud_out = single(0);
    Uq_out = single(0); 
    Us_out = single(0); 
end    
end

== matlab function TEST_IPM_2_0/INT/Motor Control/Current_PI/MATLAB Function ==
  data: Udc input; Output output; Input input
function Output = Saturation(Udc,Input)
if(Input >= Udc/sqrt(3))
    Output = Udc/sqrt(3);
elseif(Input <= -Udc/sqrt(3))
    Output = -Udc/sqrt(3);
else
    Output = Input;
end

== matlab function TEST_IPM_2_0/INT/Motor Control/TorqueMode/Current_PI1/PID_Iq/MATLAB Function ==
  data: Udc input; Output output; Input input
function Output = Saturation(Udc,Input)
if(Input >= Udc/sqrt(3))
    Output = Udc/sqrt(3);
elseif(Input <= -Udc/sqrt(3))
    Output = -Udc/sqrt(3);
else
    Output = Input;
end

== matlab function TEST_IPM_2_0/INT/Motor Control/TorqueMode/Current_PI1/PID_Iq/MATLAB Function1 ==
  data: Udc input; Output output; Input input
function Output = Saturation(Udc,Input)
if(Input >= Udc/sqrt(3))
    Output = Udc/sqrt(3);
elseif(Input <= -Udc/sqrt(3))
    Output = -Udc/sqrt(3);
else
    Output = Input;
end

== matlab function TEST_IPM_2_0/INT/Motor Control/SVPWM/MATLAB Function ==
  data: alpha input; ta output; beta input; tb output; tc output
function [ta,tb,tc] = SVPWM(alpha,beta)

temp1=beta;
temp2=0.5*beta+0.86603*alpha;
temp3=temp2-temp1;

VecSector=3;
if(temp2>0)
    VecSector=VecSector-1;
end
if(temp3>0)
    VecSector=VecSector-1;
end
if(temp1<0)
    VecSector=7-VecSector;
end

switch VecSector
    case 1
        ta=temp2;
        tb=temp1-temp3;
        tc=-temp2;
    case 2
        ta=temp3+temp2;
        tb=temp1;
        tc=-temp1;
    case 3
        ta=temp3;
        tb=-temp3;
        tc=-(temp1+temp2);
    case 4
        ta=temp2;
        tb=temp1-temp3;
        tc=-temp2;
    case 5
        ta=temp3+temp2;
        tb=temp1;
        tc=-temp1;
    case 6
        ta=temp3;
        tb=-temp3;
        tc=-(temp1+temp2);
    otherwise
        ta=single(0.5);
        tb=single(0.5);
        tc=single(0.5);
end

== matlab function TEST_IPM_2_0/SpeedREF/Subsystem1/MATLAB Function ==
  data: Target input single; Output output; Step input single; LastOutput input single; STOP data_store_memory
function Output = RAMPCONTROL(Target,Step,LastOutput)
global STOP
if(LastOutput <= Target)
    Temp = LastOutput + Step;
else
    Temp = LastOutput - Step;
end
if (abs(Temp - Target) <= Step * 2)
    Temp = Target;
end
if(STOP ~= uint16(0))
    Temp = single(0);
end
    Output = Temp;
    
end

== matlab function TEST_IPM_2_0/INT/Motor Control/Current_PI/RealVoltageCompesation /MATLAB Function ==
  data: I input; Uerror output; K input; Udead input
function Uerror = VSIComp(I,K,Udead)
% Uerror = single(2) * Udead * (single(1)/(single(1) + exp(-K*I))-single(0.5));
Uerror = Udead * atan( I * K ) /(single(pi) * single(0.5));
end

== matlab function TEST_IPM_2_0/INT/Motor Control/Current_PI/RealVoltageCompesation /MATLAB Function1 ==
  data: I input; Uerror output; K input; Udead input
function Uerror = VSIComp(I,K,Udead)
% Uerror = single(2) * Udead * (single(1)/(single(1) + exp(-K*I))-single(0.5));
Uerror = Udead * atan( I * K ) /(single(pi) * single(0.5));
end

== matlab function TEST_IPM_2_0/INT/Motor Control/Current_PI/RealVoltageCompesation /MATLAB Function2 ==
  data: I input; Uerror output; K input; Udead input
function Uerror = VSIComp(I,K,Udead)
% Uerror = single(2) * Udead * (single(1)/(single(1) + exp(-K*I))-single(0.5));
Uerror = Udead * atan( I * K ) /(single(pi) * single(0.5));
end

== matlab function TEST_IPM_2_0/INT/Motor Control/Current_PI/MATLAB Function2 ==
  data: Udc input; Output output; Input input
function Output = Saturation(Udc,Input)
if(Input >= Udc/sqrt(3))
    Output = Udc/sqrt(3);
elseif(Input <= -Udc/sqrt(3))
    Output = -Udc/sqrt(3);
else
    Output = Input;
end

== matlab function TEST_IPM_2_0/BufferOut/MATLAB Function ==
  data: ArrayId_REF data_store_memory; ArrayId_FBK data_store_memory; ArrayIq_REF data_store_memory; ArrayIq_FBK data_store_memory; ArrayUdComP data_store_memory; ArrayUqComP data_store_memory; ArrayTheta data_store_memory; BufferOutId_REF data_store_memory; BufferOutId_FBK data_store_memory; BufferOutUdComP data_store_memory; BufferOutIq_REF data_store_memory; BufferOutIq_FBK data_store_memory; BufferOutUqComP data_store_memory; BufferOutTheta data_store_memory; BufferFlag data_store_memory
function BufferOut
global ArrayId_REF ArrayId_FBK ArrayUdComP 
global ArrayIq_REF ArrayIq_FBK ArrayUqComP
global ArrayTheta
global BufferFlag    
global BufferOutId_REF BufferOutId_FBK BufferOutUdComP
global BufferOutIq_REF BufferOutIq_FBK BufferOutUqComP
global BufferOutTheta
persistent count_out switch_count;

if isempty(count_out)
    count_out =uint16(1);
end
if isempty(switch_count)
    switch_count =uint16(1);
end

if(BufferFlag == 0)
    BufferOutId_REF = single(0);
    BufferOutId_FBK = single(0);
    BufferOutUdComP = single(0);
    BufferOutIq_REF = single(0);
    BufferOutIq_FBK = single(0);
    BufferOutUqComP = single(0);
    BufferOutTheta  = single(0);
else
    if(count_out <= 500)
        switch switch_count
            case 1
                BufferOutId_REF = ArrayId_REF(count_out);
                switch_count = uint16(2);
            case 2
                BufferOutId_FBK = ArrayId_FBK(count_out);
                switch_count = uint16(3);
            case 3
                BufferOutUdComP = ArrayUdComP(count_out);
                switch_count = uint16(4);
            case 4
                BufferOutIq_REF = ArrayIq_REF(count_out);
                switch_count = uint16(5);
            case 5
                BufferOutIq_FBK = ArrayIq_FBK(count_out);
                switch_count = uint16(6);
            case 6
                BufferOutUqComP = ArrayUqComP(count_out);
                switch_count = uint16(7);
            case 7
                BufferOutTheta  =  ArrayTheta(count_out);
                switch_count = uint16(1);
                count_out = count_out + uint16(1);
        end
    else
        BufferOutId_REF = single(0);
        BufferOutId_FBK = single(0);
        BufferOutUdComP = single(0);
        BufferOutIq_REF = single(0);
        BufferOutIq_FBK = single(0);
        BufferOutUqComP = single(0);
        BufferOutTheta  = single(0);   
        count_out = uint16(1);
        BufferFlag = uint16(0);
    end
end    
    
end
